simulink model "airbag"  (R2015b)
settings: Solver=FixedStepAuto  StartTime=0.0  StopTime=inf  FixedStep=0.1  RelTol=1e-3
settings Model: Creator=scco1019  LastModifiedBy=scco1019

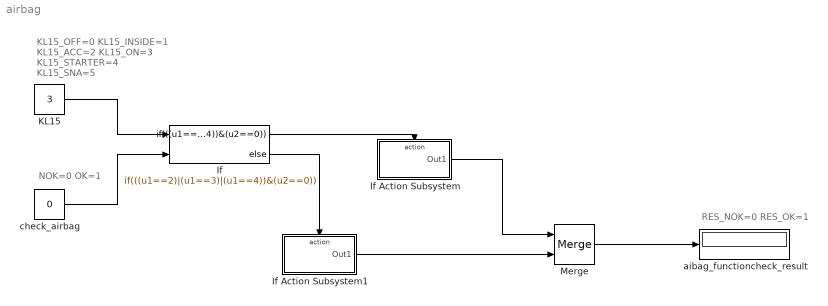
== system airbag ==
  note: RES_NOK=0
      | RES_OK=1
  note: NOK=0
      | OK=1
  note: KL15_OFF=0
      | KL15_INSIDE=1
      | KL15_ACC=2
      | KL15_ON=3
      | KL15_STARTER=4
      | KL15_SNA=5
  If : If  NumInputs=2  IfExpression=((u1==2)|(u1==3)|(u1==4))&(u2==0)
  If Action Subsystem : Subsystem  TreatAsAtomicUnit=on
  If Action Subsystem1 : Subsystem  TreatAsAtomicUnit=on
  "KL15 " : Constant  Value=3
  Merge : Merge
  aibag_functioncheck_result : Display
  check_airbag : Constant  Value=0
  wires:
  "KL15 "/1 -> If/1
  check_airbag/1 -> If/2
  If/1 -> If Action Subsystem/Action
  If/2 -> If Action Subsystem1/Action
  If Action Subsystem/1(Out1) -> Merge/1
  If Action Subsystem1/1(Out1) -> Merge/2
  Merge/1 -> aibag_functioncheck_result/1

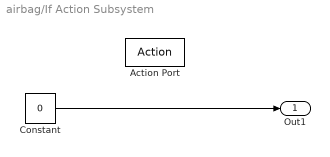
== system airbag/If Action Subsystem ==
  Action Port : ActionPort  ActionType=then
  Constant : Constant  Value=0
  Out1 : Outport
  wires:
  Constant/1 -> Out1/1

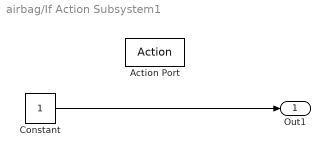
== system airbag/If Action Subsystem1 ==
  Action Port : ActionPort  ActionType=else
  Constant : Constant
  Out1 : Outport
  wires:
  Constant/1 -> Out1/1
